simulink model "simu_22a"  (R2022a)
settings: Solver=VariableStepAuto  StartTime=0.0  StopTime=5  RelTol=1e-3
settings Model: Creator=zhang  LastModifiedBy=psp_dada
settings ModelReferenceCC: EnableRefExpFcnMdlSchedulingChecks=off
settings RTWCC: Description=Generic Real-Time Target
settings ConfigComp: CovBoundaryAbsTol=1.0e-5

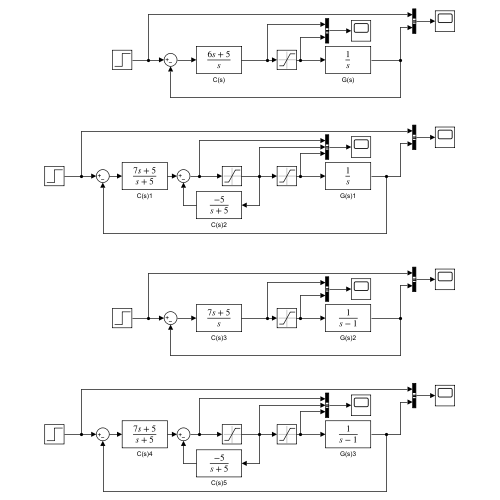
[thumbnail: Simulink's stored preview of the top-level diagram]
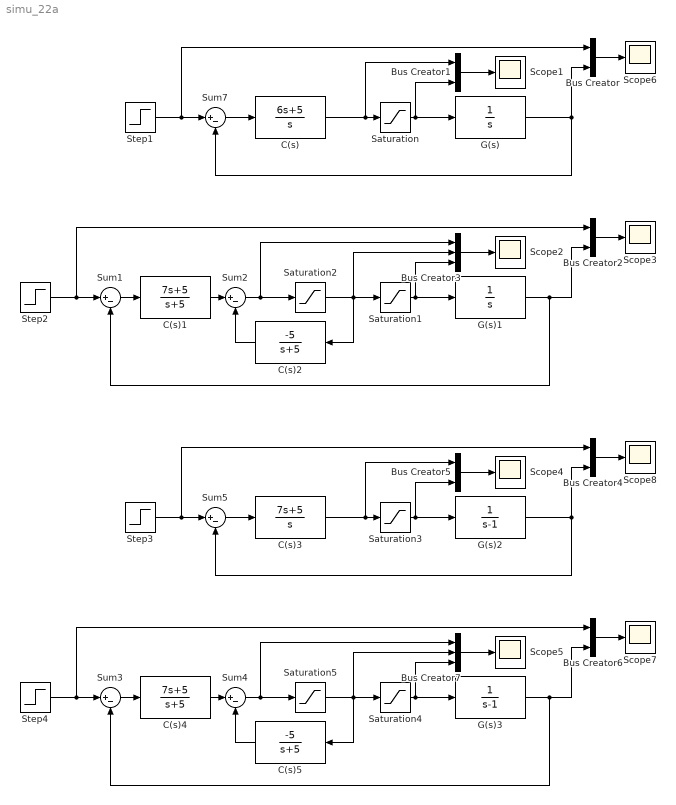
== system simu_22a ==
  Bus Creator{,1..2,4..6} (6 alike) : BusCreator  Inputs=2
  Bus Creator3 : BusCreator  Inputs=3
  Bus Creator7 : BusCreator  Inputs=3
  C(s) : TransferFcn  Numerator=[6 5]  Denominator=[1 0]
  C(s)1 : TransferFcn  Numerator=[7 5]  Denominator=[1 5]
  C(s)2 : TransferFcn  Numerator=[-5]  Denominator=[1 5]
  C(s)3 : TransferFcn  Numerator=[7 5]  Denominator=[1 0]
  C(s)4 : TransferFcn  Numerator=[7 5]  Denominator=[1 5]
  C(s)5 : TransferFcn  Numerator=[-5]  Denominator=[1 5]
  G(s) : TransferFcn  Denominator=[1 0]
  G(s)1 : TransferFcn  Denominator=[1 0]
  G(s)2 : TransferFcn  Denominator=[1 -1]
  G(s)3 : TransferFcn  Denominator=[1 -1]
  Saturation{,1..5} (6 alike) : Saturate  UpperLimit=1  LowerLimit=-1
  Scope{1..8} (8 alike) : Scope
  Step1 : Step  After=4  SampleTime=0
  Step2 : Step  After=4  SampleTime=0
  Step3 : Step  After=.8  SampleTime=0
  Step4 : Step  After=0.8  SampleTime=0
  Sum{1..5,7} (6 alike) : Sum  Inputs=|+-
  wires:
  G(s)/1 -> Bus Creator/2, Sum7/2
  Saturation/1 -> Bus Creator1/2, G(s)/1
  C(s)/1 -> Bus Creator1/1, Saturation/1
  Sum7/1 -> C(s)/1
  Step1/1 -> Bus Creator/1, Sum7/1
  Bus Creator/1 -> Scope6/1
  Bus Creator1/1 -> Scope1/1
  Bus Creator3/1 -> Scope2/1
  Saturation2/1 -> Bus Creator3/2, C(s)2/1, Saturation1/1
  Step2/1 -> Bus Creator2/1, Sum1/1
  Bus Creator2/1 -> Scope3/1
  Sum1/1 -> C(s)1/1
  Saturation1/1 -> Bus Creator3/3, G(s)1/1
  G(s)1/1 -> Bus Creator2/2, Sum1/2
  C(s)1/1 -> Sum2/1
  C(s)2/1 -> Sum2/2
  Sum2/1 -> Bus Creator3/1, Saturation2/1
  C(s)5/1 -> Sum4/2
  Bus Creator5/1 -> Scope4/1
  G(s)3/1 -> Bus Creator6/2, Sum3/2
  Saturation4/1 -> Bus Creator7/3, G(s)3/1
  Step4/1 -> Bus Creator6/1, Sum3/1
  Bus Creator7/1 -> Scope5/1
  Step3/1 -> Bus Creator4/1, Sum5/1
  C(s)3/1 -> Bus Creator5/1, Saturation3/1
  Saturation3/1 -> Bus Creator5/2, G(s)2/1
  Sum4/1 -> Bus Creator7/1, Saturation5/1
  Bus Creator4/1 -> Scope8/1
  Bus Creator6/1 -> Scope7/1
  Saturation5/1 -> Bus Creator7/2, C(s)5/1, Saturation4/1
  Sum3/1 -> C(s)4/1
  C(s)4/1 -> Sum4/1
  Sum5/1 -> C(s)3/1
  G(s)2/1 -> Bus Creator4/2, Sum5/2
